simulink model "power_machines_sync"  (R2014a)
settings: Solver=ode23tb  SolverMode=SingleTasking  StartTime=0.0  StopTime=90  RelTol=1e-4
undefined symbols (not defined in the file or in its folder): D1, Delta
libraries: powerlib x11, sps_avr x7, sdolib x2, powerlib_meascontrol x2, simulink x1
Description:
  | Copyright 2008-2014 The MathWorks, Inc.
settings Model: FPTRunName=Active  ExtModeTrigMode=oneshot  ExtModeArmWhenConnect=off  ExtModeAutoUpdateStatusClock=off  Creator=MathWorks  LastModifiedBy=jdlara
settings SolverCC: ZeroCrossAlgorithm=Adaptive
settings DataIOCC: LimitDataPoints=off  SignalLoggingSaveFormat=ModelDataLogs  SignalLoggingName=sigsOut  OutputTimes=[0:1/20:10]
settings OptimizationCC: BlockReduction=off  BooleanDataType=off  ExpressionDepthLimit=2147483647  InitFltsAndDblsToZero=on  EfficientMapNaN2IntZero=off
settings DebuggingCC: UnderspecifiedInitializationDetection=Classic  CheckExecutionContextPreStartOutputMsg=on  CheckExecutionContextRuntimeOutputMsg=on  SignalResolutionControl=TryResolveAllWithWarning  IgnoredZcDiagnostic=none  SolverPrmCheckMsg=none  MultiTaskDSMMsg=warning  MultiTaskCondExecSysMsg=none  SigSpecEnsureSampleTimeMsg=none  FcnCallInpInsideContextMsg=UseLocalSettings  UnconnectedInputMsg=none  UnconnectedOutputMsg=none  UnconnectedLineMsg=none  StateNameClashWarn=warning
settings HardwareCC: ProdHWDeviceType=Specified  TargetUnknown=on
settings RTWCC: IncludeERTFirstTime=on
settings CodeAppCC: IgnoreCustomStorageClasses=off
settings GRTTargetCC: TargetFcnLib=ansi_tfl_tmw.mat  CombineOutputUpdateFcns=off  GRTInterface=on

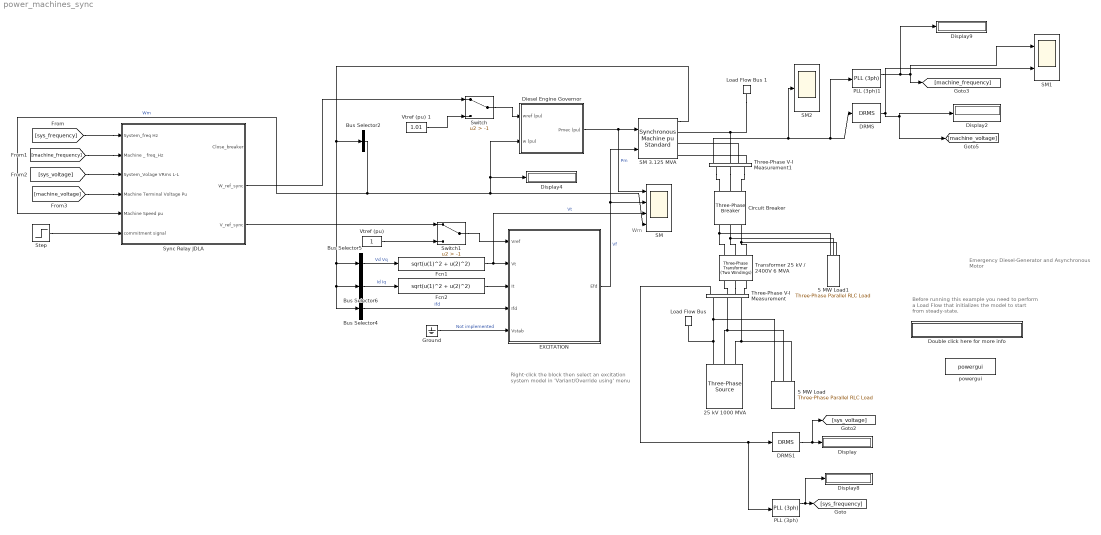
== system power_machines_sync ==
  note: Emergency Diesel-Generator
      | and Asynchronous Motor
  note: Right-click the block then select
      | an excitation system model in
      | 'Variant/Override using' menu
  note: Wm
  note: Before running this example you
      | need to perform a Load Flow that
      | initializes the model to start from
      | steady-state.
  25 kV 1000 MVA : powerlib/Electrical Sources/Three-Phase Source  Voltage=(25000)*1  PhaseAngle=2.1395e-05  Frequency=60  InternalConnection=Yg  SpecifyImpedance=on  Resistance=25^2/1000/10  Inductance=25^2/1000/377  ShortCircuitLevel=1000e6  BaseVoltage=25e3  XRratio=10  BusType=swing  Pref=0  Qref=0  Qmin=-Inf  Qmax=Inf
  5 MW Load : powerlib/Elements/Three-Phase Parallel RLC Load  LConnTagsString=A|B|C  Configuration=Y (grounded)  NominalVoltage=25e3  NominalFrequency=60  ActivePower=5e+006  InductivePower=0  CapacitivePower=0  Measurements=None  LoadType=constant Z
  5 MW Load1 : powerlib/Elements/Three-Phase Parallel RLC Load  LConnTagsString=A|B|C  Configuration=Y (grounded)  NominalVoltage=2400  NominalFrequency=60  ActivePower=5e+99  InductivePower=0  CapacitivePower=0  Measurements=None  LoadType=constant Z
  Bus Selector2 : BusSelector  OutputSignals="Mechanical.Rotor speed  wm  (pu)"  OutputAsBus=on
  Bus Selector4 : BusSelector  OutputSignals="dq0 components.Field current  ifd (pu)"  OutputAsBus=on
  Bus Selector5 : BusSelector  OutputSignals="dq0 components.Stator voltage  vd (pu),dq0 components.Stator voltage  vq (pu)"  OutputAsBus=on
  Bus Selector6 : BusSelector  OutputSignals="dq0 components.Stator current  id (pu),dq0 components.Stator current  iq (pu)"  OutputAsBus=on
  Circuit Breaker : powerlib/Elements/Three-Phase Breaker  InitialState=open  SwitchA=on  SwitchB=on  SwitchC=on  SwitchTimes=[600]  External=off  BreakerResistance=0.01  SnubberResistance=1e5  SnubberCapacitance=inf  Measurements=None
      settings: AttributesFormatString=\n
  DRMS : sdolib/RMS Blocks/DRMS  Ts=0.00167
  DRMS1 : sdolib/RMS Blocks/DRMS  Ts=0.00167
  Diesel Engine Governor : Subsystem  mask(Diesel Engine & Governor){K=40, Tr=[0.01 0.02 0.2], Ta=[0.25 0.009 0.0384], Tlim=[0 1.1], Td=0.024, Pm0=0}
      mask prompts: K "Regulator gain K:"; Tr "Regulator time constants [T1 T2 T3 ] (s) :"; Ta "Actuator time constants [T4 T5 T6] (s) :"; Tlim "Torque limits [Tmin Tmax] (pu) :"; Td "Engine time delay Td (s) :"; Pm0 "Initial value of mechanical power  Pm0 (pu) :"
      mask help:
      | This block implements a diesel engine and governor system:
      | 1st and 2nd inputs: Desired and actual speed (pu)
      | Output: Diesel engine mechanical power.Motor inertia should be combined with generator.
      | Controller transfer function:
      |      Hc=K.(1+T3.s)/(1+T1.s+T1.T2.s^2)
      | Actuator transfer function :
      |      Ha= (1+T4.s) / [ (s (1+T5.s)(1+T6.s) ]
      | Motor :
      |      Time delay Td
      |
      | (See reference in Tutorial Session 5)
  Display{,2,4,8..9} (5 alike) : Display
      Display9 settings: Decimation=11
  Double click here for more info : Subsystem
      settings: OpenFcn=showdemo(bdroot(gcb))
      mask Display: disp('Double-click here for more information')
  EXCITATION : Subsystem  Variant=on  OverrideUsingVariant=Variant1
      settings: AttributesFormatString=%<BlockChoice>
  Fcn1 : Fcn  Expr=sqrt(u(1)^2 + u(2)^2)
  Fcn2 : Fcn  Expr=sqrt(u(1)^2 + u(2)^2)
  Ground : Ground
  Load Flow Bus 1 : powerlib/Measurements/Load Flow Bus  LConnTagsString=a  ID=B2  Vbase=2.4e3  Vref=1  Vangle=0  VLF=1  angleLF=-31.89
      settings: AttributesFormatString=%<ID>\n%<Vbase>V\n%<VLF>pu\n%<angleLF>deg.
  Load Flow Bus : powerlib/Measurements/Load Flow Bus  LConnTagsString=a  ID=B1  Vbase=25e3  Vref=0.999364  Vangle=-0.4332  VLF=0.9994  angleLF=-0.4332
      settings: AttributesFormatString=%<ID>\n%<Vbase>V\n%<VLF>pu\n%<angleLF>deg.
  PLL (3ph) : powerlib_meascontrol/PLL/PLL (3ph)  Fmin=45  Par_Init=[0, 60]  ParK=[180, 3200, 1]  TcD=1e-4  MaxRateChangeFreq=12  FilterCutOffFreq=25  Ts=0  AGC=on
  PLL (3ph)1 : powerlib_meascontrol/PLL/PLL (3ph)  Fmin=45  Par_Init=[0, 10]  ParK=[180, 3200, 1]  TcD=1e-4  MaxRateChangeFreq=12  FilterCutOffFreq=25  Ts=0  AGC=on
  SM : Scope  NumInputPorts=4
      settings: ShowLegends=on  TimeRange=10  YMin=0.04675~4.9495~0.248~0.99762  YMax=0.05~4.9535~0.259~0.99773  SaveName=Pmec_SM1  DataFormat=Structure  Decimation=10
  SM 3.125 MVA : powerlib/Machines/Synchronous Machine pu Standard  PresetModel=No  MechanicalLoad=Mechanical power Pm  ShowDetailedParameters=on  RotorType=Salient-pole  Units=per unit standard parameters  MeasurementBus=off  NominalParameters="[ 3.125e6  2400  60]"  Reactances1=[ 31 32 33 34 35 36 37 ]  Reactances2=[ 1.56, 0.296, 0.177, 1.06, 0.177, 0.052 ]  dAxisTimeConstants=Short-circuit  qAxisTimeConstants=Open-circuit  TimeConstants1=[]  TimeConstants2=[]  TimeConstants3=[]  TimeConstants4=[]  TimeConstants5=[ 3.7, 0.05, 0.05 ]  TimeConstants6=[ 8.0, 0.03, 0.3371, 0.0295 ]  TimeConstants7=[0.024 0.006 0.006]  TimeConstants8=[]  StatorResistance=0.0036  Mechanical="[ 1.07  0.05 2]"  PolePairs=2  InitialConditions=[-99.9 0 0 0 0 0 0 0 0]  SetSaturation=off  Saturation=[0.211 0.418 1.0 1.25 1.72 3.35 ;0.25 0.50 1.0 1.1 1.2 1.4]  LoadFlowParameters=[1 0 0 0]  TsPowergui=0  TsBlock=-1  IterativeModel=Forward Euler  BusType=PV  Pref=0  Qref=0  Qmin=-Inf  Qmax=Inf  PLF=0  QLF=0
      settings: AttributesFormatString=\n\n
  SM1 : Scope  NumInputPorts=2
      settings: ShowLegends=on  TimeRange=4.5  YMin=9.5~2.68e-52  YMax=10.5~2.7275e-52  SaveName=Pmec_SM  DataFormat=Structure  Decimation=10  SampleInput=on
  SM2 : Scope
      settings: ShowLegends=on  TimeRange=10  YMin=-8e-05  YMax=8e-05  SaveName=Pmec_SM2  DataFormat=Structure  Decimation=10  SampleInput=on
  Step : Step  Time=0.4  SampleTime=0
  Switch : Switch  Criteria=u2 > Threshold  Threshold=-1
  Switch1 : Switch  Criteria=u2 > Threshold  Threshold=-1
  Sync Relay JDLA : Subsystem  mask{BaseFrequency=60, BaseRMSVoltageSystem=1, avr_speed_ini=0.8}
      mask prompts: BaseFrequency "Base Frequency"; BaseRMSVoltageSystem "Base Line-Line RMS voltage"; avr_speed_ini "AVR speed threshold"
      mask init:
      | BaseFrequency=60;
      | BaseRMSVoltage=25000;
      | avr_speed_ini=0.8;
  Three-Phase V-I Measurement : powerlib/Measurements/Three-Phase V-I Measurement  VoltageMeasurement=phase-to-phase  SetLabelV=off  LabelV=Vabc  Vpu=off  VpuLL=on  CurrentMeasurement=yes  SetLabelI=off  LabelI=Iabc  Ipu=on  Pbase=100e6  Vbase=(25000)*1/sqrt(2)  OutputType=Complex  PhasorSimulation=off  PSBequivalent=0
  Three-Phase V-I Measurement1 : powerlib/Measurements/Three-Phase V-I Measurement  VoltageMeasurement=phase-to-phase  SetLabelV=off  LabelV=Vabc  Vpu=off  VpuLL=on  CurrentMeasurement=yes  SetLabelI=off  LabelI=Iabc  Ipu=on  Pbase=100e6  Vbase=(2400)*1/sqrt(2)  OutputType=Complex  PhasorSimulation=off  PSBequivalent=0
  Transformer 25 kV / 2400V 6 MVA : powerlib/Elements/Three-Phase Transformer (Two Windings)  Winding1Connection=Yg  UNITS=pu  NominalPower=[ 6e6 , 60 ]  Winding1=[ 25e3 , 0.0015 , 0.03]  Winding2Connection=Delta (D1)  Winding2=[ 2.4e3 , 0.0015 , 0.03 ]  SetSaturation=off  Rm=200  Lm=200  Saturation="[ 0,0  ;  0.005,1.2  ;  1.0,1.4 ]"  Hysteresis=off  DataFile='hysteresis'  SetInitialFlux=off  InitialFluxes=[ 0.8 , -0.8 , 0.7 ]  Measurements=None  MoreParameters=off  BreakLoop=off  DataType=off  TransfoNumber=0
  "Vtref (pu) " : Constant
  Vtref (pu) 1 : Constant  Value=1.01
  powergui : powerlib/powergui  Priority=2  SimulationMode=Continuous  SolverType=Tustin  SampleTime=50e-6  frequency=60  SPID=off  DisableSnubberDevices=off  DisableRonSwitches=off  DisableVfSwitches=off  SwTol=0  Interpol=off  DisplayEquations=off  Ts=0  methode=off  frequencyindice=60  Pbase=1e6  ErrMax=0.0001  Iterations=50  UnitsV=kV  UnitsW=MW  FunctionMessages=off  echomessages=off  HookPort=off  EnableUseOfTLC=off  x0status=blocks  RestoreLinks=warning  ResistiveCurrentMeasurement=off  Frange=logspace(0,3,50)  Ylog=off  Xlog=off  ShowGrid=off  save=off  variable=ZData  structure=0  ZoomFFT=on  StartTime=0.0  cycles=2  DisplayStyle=off  fundamental=60  FreqAxis=off  MaxFrequency=1000  frequencyindicesteady=1  RmsSteady=1  display=off
  wires:
  Diesel Engine Governor/1(Pmec (pu)) -> SM/1, SM 3.125 MVA/1  "Pm"
  Fcn2/1 -> EXCITATION/3(It)
  Bus Selector4/1 -> EXCITATION/4(Ifd)  "Ifd"
  Bus Selector6/1 -> Fcn2/1  "Id Iq"
  Ground/1 -> EXCITATION/5(Vstab)  "Not implemented"
  Bus Selector5/1 -> Fcn1/1  "Vd Vq"
  Fcn1/1 -> EXCITATION/2(Vt), SM/3  "Vt"
  EXCITATION/1(Efd) -> SM 3.125 MVA/2, SM/2  "Vf"
  SM 3.125 MVA/1 -> Bus Selector2/1, Bus Selector5/1, Bus Selector6/1, Bus Selector4/1
  DRMS1/1 -> [sys_voltage], Display/1
  Three-Phase V-I Measurement/1 -> DRMS1/1, PLL (3ph)/1
  Bus Selector2/1 -> Display4/1, Diesel Engine Governor/2(w (pu)), SM/4, Sync Relay JDLA/5(Machine Speed pu)  "Wm"
  Switch/1 -> Diesel Engine Governor/1(wref (pu))
  Switch1/1 -> EXCITATION/1(Vref)
  "Vtref (pu) "/1 -> Switch1/3
  PLL (3ph)/1 -> Display8/1, [sys_frequency]
  Three-Phase V-I Measurement1/1 -> SM2/1, DRMS/1, PLL (3ph)1/1
  PLL (3ph)1/1 -> Display9/1, SM1/1, [machine_frequency]
  DRMS/1 -> [machine_voltage], Display2/1, SM1/2
  Sync Relay JDLA/3(V_ref_sync) -> Switch1/1
  Sync Relay JDLA/2(W_ref_sync) -> Switch/1
  [sys_frequency] -> Sync Relay JDLA/1(System_freq Hz)
  [machine_frequency] -> Sync Relay JDLA/2(Machine _ freq_Hz)
  [sys_voltage] -> Sync Relay JDLA/3(System_Volage VRms L-L)
  [machine_voltage] -> Sync Relay JDLA/4(Machine Terminal Voltage Pu)
  Step/1 -> Sync Relay JDLA/6(commitment signal)
  Vtref (pu) 1/1 -> Switch/3
  connections:
  Three-Phase V-I Measurement1/RConn2 -- SM 3.125 MVA/RConn2
  Load Flow Bus 1/LConn1 -- Three-Phase V-I Measurement1/RConn1 -- SM 3.125 MVA/RConn1
  Three-Phase V-I Measurement1/RConn3 -- SM 3.125 MVA/RConn3
  25 kV 1000 MVA/RConn1 -- Three-Phase V-I Measurement/LConn1 -- 5 MW Load/LConn1 -- Load Flow Bus/LConn1
  25 kV 1000 MVA/RConn2 -- Three-Phase V-I Measurement/LConn2 -- 5 MW Load/LConn2
  5 MW Load/LConn3 -- 25 kV 1000 MVA/RConn3 -- Three-Phase V-I Measurement/LConn3
  Transformer 25 kV / 2400V 6 MVA/LConn2 -- Three-Phase V-I Measurement/RConn2
  Transformer 25 kV / 2400V 6 MVA/LConn3 -- Three-Phase V-I Measurement/RConn3
  Transformer 25 kV / 2400V 6 MVA/LConn1 -- Three-Phase V-I Measurement/RConn1
  Circuit Breaker/LConn3 -- 5 MW Load1/LConn3 -- Transformer 25 kV / 2400V 6 MVA/RConn3
  Circuit Breaker/LConn2 -- 5 MW Load1/LConn2 -- Transformer 25 kV / 2400V 6 MVA/RConn2
  Circuit Breaker/LConn1 -- 5 MW Load1/LConn1 -- Transformer 25 kV / 2400V 6 MVA/RConn1
  Three-Phase V-I Measurement1/LConn1 -- Circuit Breaker/RConn1
  Three-Phase V-I Measurement1/LConn2 -- Circuit Breaker/RConn2
  Three-Phase V-I Measurement1/LConn3 -- Circuit Breaker/RConn3

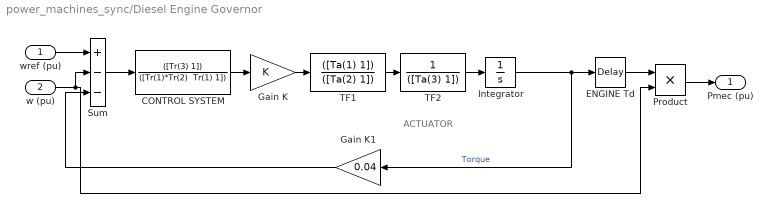
== system power_machines_sync/Diesel Engine Governor ==
  note: ACTUATOR
  wref (pu) : Inport
  w (pu) : Inport  Port=2
  CONTROL SYSTEM : TransferFcn  Numerator=([Tr(3) 1])  Denominator="([Tr(1)*Tr(2)  Tr(1) 1])"
  ENGINE Td : TransportDelay  DelayTime=Td  InitialOutput=Pm0
  Gain K : Gain  Gain=K  SaturateOnIntegerOverflow=on  OutDataTypeStr=Inherit: Same as input  ParamDataTypeStr=Inherit: Same as input
  Gain K1 : Gain  Gain=0.04  SaturateOnIntegerOverflow=on  OutDataTypeStr=Inherit: Same as input  ParamDataTypeStr=Inherit: Same as input
  Integrator : Integrator  InitialCondition=Pm0  LimitOutput=on  UpperSaturationLimit=Tlim(2)  LowerSaturationLimit=Tlim(1)
  Product : Product  SaturateOnIntegerOverflow=on  InputSameDT=on  OutDataTypeStr=Inherit: Same as first input
  Sum : Sum  Inputs=+--  SaturateOnIntegerOverflow=on  InputSameDT=on  OutDataTypeStr=Inherit: Same as first input
  TF1 : TransferFcn  Numerator=([Ta(1) 1])  Denominator=([Ta(2) 1])
  TF2 : TransferFcn  Numerator=1  Denominator=([Ta(3) 1])
  Pmec (pu) : Outport  InitialOutput=0
  wires:
  Integrator/1 -> Gain K1/1, ENGINE Td/1  "Torque"
  TF2/1 -> Integrator/1
  Product/1 -> Pmec (pu)/1
  wref (pu)/1 -> Sum/1
  ENGINE Td/1 -> Product/1
  w (pu)/1 -> Sum/2, Product/2
  TF1/1 -> TF2/1
  CONTROL SYSTEM/1 -> Gain K/1
  Sum/1 -> CONTROL SYSTEM/1
  Gain K/1 -> TF1/1
  Gain K1/1 -> Sum/3

== system power_machines_sync/Double click here for more info ==

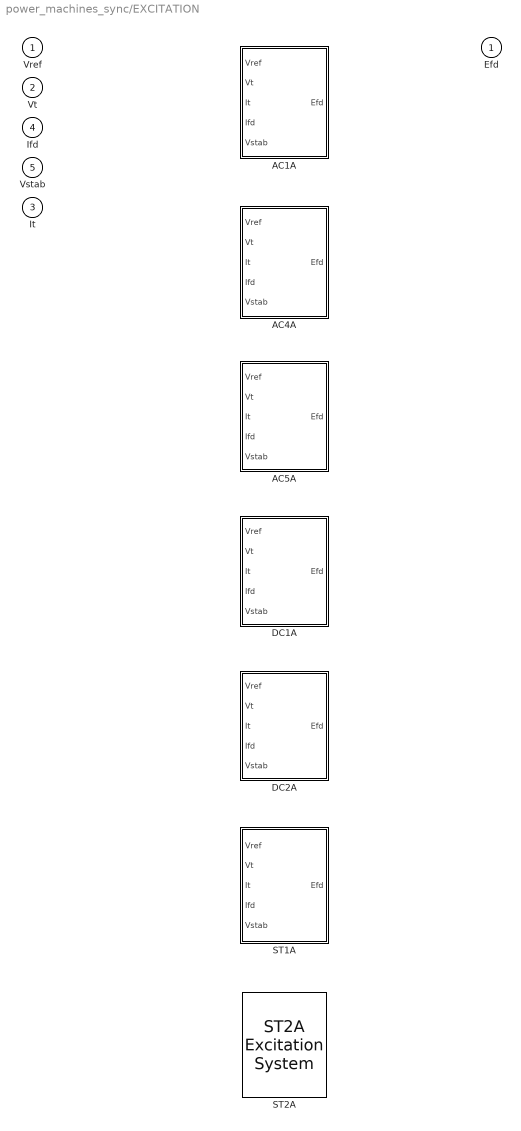
== system power_machines_sync/EXCITATION ==
  Vref : Inport
  Vt : Inport  Port=2
  It : Inport  Port=3
  Ifd : Inport  Port=4
  Vstab : Inport  Port=5
  AC1A : Subsystem  VariantControl=Variant1
  AC4A : Subsystem  VariantControl=Variant2
  AC5A : Subsystem  VariantControl=Variant3
  DC1A : Subsystem  VariantControl=Variant4
  DC2A : Subsystem  VariantControl=Variant5
  ST1A : Subsystem  VariantControl=Variant6
  ST2A : sps_avr/ST2A Excitation System  VariantControl=Variant7  Tr=20e-3  KaTa=[120 0.15]  VRminmax=[0 1.0]  KfTf=[0.05 1.0]  KeTe=[1.0 0.5]  KI=8.0  Kp=4.88  Xd=1.56  Kc=1.82  v0=[1,1.42734]  I0=0.2739  TsBlock=-2
  Efd : Outport

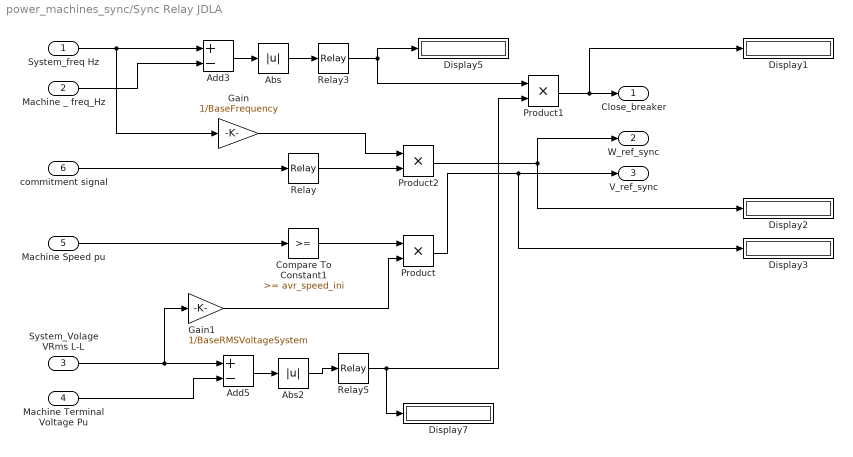
== system power_machines_sync/Sync Relay JDLA ==
  System_freq Hz : Inport
  Machine _ freq_Hz : Inport  Port=2
  System_Volage VRms L-L : Inport  Port=3
  Machine Terminal Voltage Pu : Inport  Port=4
  Machine Speed pu : Inport  Port=5
  commitment signal : Inport  Port=6
  Abs : Abs
  Abs2 : Abs
  Add3 : Sum  Inputs=+-
  Add5 : Sum  Inputs=+-
  Compare To Constant1 : simulink/Logic and Bit Operations/Compare To Constant  relop=>=  const=avr_speed_ini  OutDataTypeStr=boolean
  Display{1..3,5,7} (5 alike) : Display
  Gain : Gain  Gain=1/BaseFrequency
  Gain1 : Gain  Gain=1/BaseRMSVoltageSystem
  Product : Product
  Product1 : Product
  Product2 : Product
  Relay : Relay  OnSwitchValue=1  OffSwitchValue=0
  Relay3 : Relay  OnSwitchValue=1  OffSwitchValue=0.15  OnOutputValue=0  OffOutputValue=1
  Relay5 : Relay  OnSwitchValue=1  OffSwitchValue=0.05  OnOutputValue=0  OffOutputValue=1
  Close_breaker : Outport
  W_ref_sync : Outport  Port=2
  V_ref_sync : Outport  Port=3
  wires:
  System_Volage VRms L-L/1 -> Gain1/1, Add5/1
  System_freq Hz/1 -> Gain/1, Add3/1
  Machine _ freq_Hz/1 -> Add3/2
  Machine Terminal Voltage Pu/1 -> Add5/2
  Relay3/1 -> Product1/1, Display5/1
  Add3/1 -> Abs/1
  Relay5/1 -> Product1/2, Display7/1
  Abs/1 -> Relay3/1
  Add5/1 -> Abs2/1
  Abs2/1 -> Relay5/1
  Gain/1 -> Product2/1
  Compare To Constant1/1 -> Product/1
  Gain1/1 -> Product/2
  Product/1 -> Display3/1, V_ref_sync/1
  Product1/1 -> Display1/1, Close_breaker/1
  Product2/1 -> W_ref_sync/1, Display2/1
  commitment signal/1 -> Relay/1
  Relay/1 -> Product2/2
  Machine Speed pu/1 -> Compare To Constant1/1

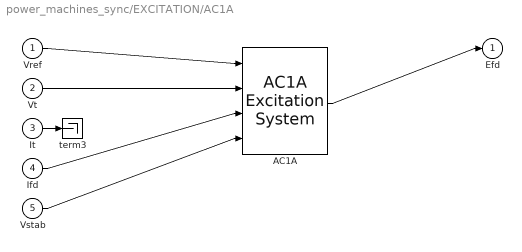
== system power_machines_sync/EXCITATION/AC1A ==
  Vref : Inport
  Vt : Inport  Port=2
  It : Inport  Port=3
  Ifd : Inport  Port=4
  Vstab : Inport  Port=5
  AC1A : sps_avr/AC1A Excitation System  Tr=20e-11  KaTa=[400 0.02]  VAminmax=[-14.5 14.5]  VRminmax=[-5.43 8.03]  KfTf=[0.03 1.0]  TbTc=[0 0]  KeTe=[1.0 0.50]  Ve12=[10.18 7.14]  SeVe12=[0.10 0.03]  Kd=0.38  Kc=0.20  v0=[0 0]  TsBlock=-2
  term3 : Terminator
  Efd : Outport
  wires:
  It/1 -> term3/1
  AC1A/1 -> Efd/1
  Vstab/1 -> AC1A/4
  Ifd/1 -> AC1A/3
  Vt/1 -> AC1A/2
  Vref/1 -> AC1A/1

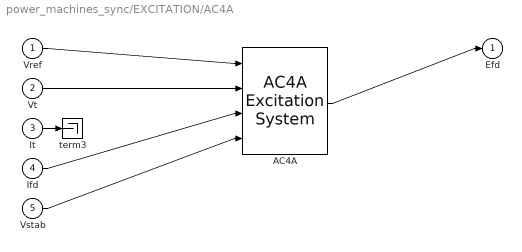
== system power_machines_sync/EXCITATION/AC4A ==
  Vref : Inport
  Vt : Inport  Port=2
  It : Inport  Port=3
  Ifd : Inport  Port=4
  Vstab : Inport  Port=5
  AC4A : sps_avr/AC4A Excitation System  Tr=20e-3  KaTa=[200 0.015]  VIminmax=[-10 10]  VRminmax=[-4.53 5.64]  TbTc=[10 1.0]  Kc=0  v0=[1,1.42734]  TsBlock=-2
  term3 : Terminator
  Efd : Outport
  wires:
  It/1 -> term3/1
  AC4A/1 -> Efd/1
  Vstab/1 -> AC4A/4
  Ifd/1 -> AC4A/3
  Vt/1 -> AC4A/2
  Vref/1 -> AC4A/1

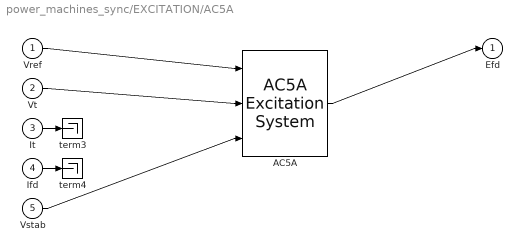
== system power_machines_sync/EXCITATION/AC5A ==
  Vref : Inport
  Vt : Inport  Port=2
  It : Inport  Port=3
  Ifd : Inport  Port=4
  Vstab : Inport  Port=5
  AC5A : sps_avr/AC5A Excitation System  Tr=20e-3  KaTa=[100 0.02]  VRminmax=[-7.3 7.3]  KfTf=[0.03 1 0 0]  KeTe=[1.0 0.02]  Efd12=[5.6 0.75*5.6]  SeEfd12=[0.86 0.5]  v0=[1,1.42734]  TsBlock=-2
  term3 : Terminator
  term4 : Terminator
  Efd : Outport
  wires:
  Ifd/1 -> term4/1
  It/1 -> term3/1
  AC5A/1 -> Efd/1
  Vstab/1 -> AC5A/3
  Vt/1 -> AC5A/2
  Vref/1 -> AC5A/1

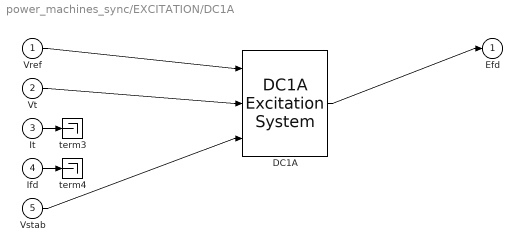
== system power_machines_sync/EXCITATION/DC1A ==
  Vref : Inport
  Vt : Inport  Port=2
  It : Inport  Port=3
  Ifd : Inport  Port=4
  Vstab : Inport  Port=5
  DC1A : sps_avr/DC1A Excitation System  Tr=20e-3  KaTa=[46 0.06]  VRminmax=[-0.9 1.0]  KfTf=[0.05 1.5]  TbTc=[0 0]  KeTe=[0.05 0.46]  Efd12=[3.1 2.3]  SeEfd12=[0.33 0.10]  v0=[1,1.42734]  TsBlock=-2
  term3 : Terminator
  term4 : Terminator
  Efd : Outport
  wires:
  Ifd/1 -> term4/1
  It/1 -> term3/1
  DC1A/1 -> Efd/1
  Vstab/1 -> DC1A/3
  Vt/1 -> DC1A/2
  Vref/1 -> DC1A/1

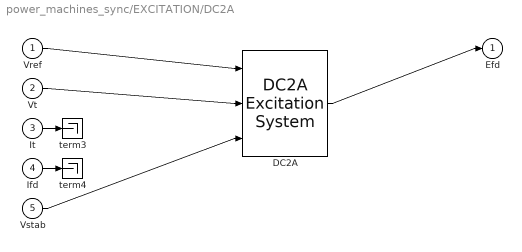
== system power_machines_sync/EXCITATION/DC2A ==
  Vref : Inport
  Vt : Inport  Port=2
  It : Inport  Port=3
  Ifd : Inport  Port=4
  Vstab : Inport  Port=5
  DC2A : sps_avr/DC2A Excitation System  Tr=20e-3  KaTa=[46 0.06]  VRminmax=[-4.9 4.95]  KfTf=[0.05 1.5]  TbTc=[0 0]  KeTe=[0.05 0.46]  Efd12=[3.05 2.29]  SeEfd12=[0.279 0.117]  v0=[1,1.42734]  TsBlock=-2
  term3 : Terminator
  term4 : Terminator
  Efd : Outport
  wires:
  Ifd/1 -> term4/1
  It/1 -> term3/1
  DC2A/1 -> Efd/1
  Vstab/1 -> DC2A/3
  Vt/1 -> DC2A/2
  Vref/1 -> DC2A/1

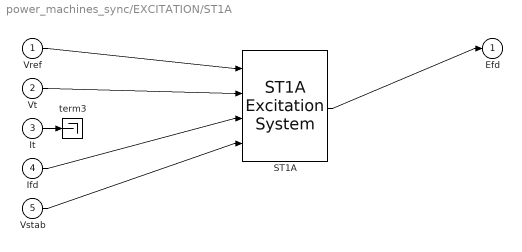
== system power_machines_sync/EXCITATION/ST1A ==
  Vref : Inport
  Vt : Inport  Port=2
  It : Inport  Port=3
  Ifd : Inport  Port=4
  Vstab : Inport  Port=5
  ST1A : sps_avr/ST1A Excitation System  Tr=20e-3  KaTa=[210 0.001]  VIminmax=[-999 999]  VAminmax=[-999 999]  VRminmax=[-6.0 6.43]  KfTf=[0.001 1]  TbTc=[0 0 0 0]  KLR=1  ILR=2  Kc=0.038  v0=[1,1.42734]  TsBlock=-2
  term3 : Terminator
  Efd : Outport
  wires:
  It/1 -> term3/1
  ST1A/1 -> Efd/1
  Vstab/1 -> ST1A/4
  Ifd/1 -> ST1A/3
  Vt/1 -> ST1A/2
  Vref/1 -> ST1A/1
